simulink model "koen_observer_pll_model"  (R2024b)
settings: Solver=FixedStepDiscrete  StartTime=0.0  StopTime=0.05  FixedStep=6.25e-05  RelTol=1e-3
PreLoadFcn:
  | FOC_TS_SEC=6.25e-05; FOC_RS_OHM=0.53; FOC_LS_H=0.0006; FOC_FLUX_WB=0.0078; FOC_FLUX_LIMIT_RATIO=1.5; FOC_OBS_PLL_KP=180; FOC_OBS_PLL_KI=6000; FOC_OBS_PLL_INTEGRAL_LIMIT=700; FOC_OBS_SPEED_LIMIT_RAD_S=1200; FOC_OBS_SPEED_FILTER_ALPHA=0.2; FOC_OBS_THETA_COMP_RAD=2.7239; FOC_TWO_PI=6.283185307179586;
settings Model: Creator=10095  LastModifiedBy=10095

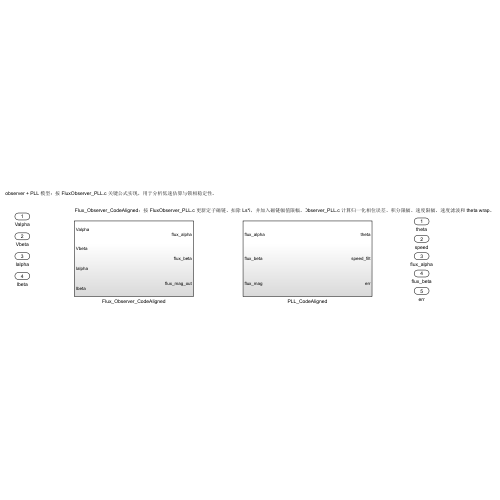
[thumbnail: Simulink's stored preview of the top-level diagram]
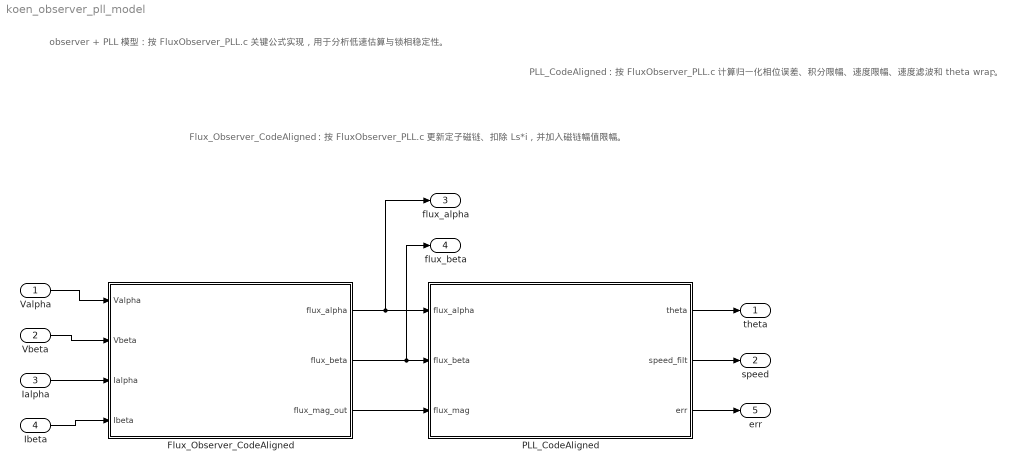
== system koen_observer_pll_model ==
  note: Flux_Observer_CodeAligned：按 FluxObserver_PLL.c 更新定子磁链、扣除 Ls*i，并加入磁链幅值限幅。
  note: PLL_CodeAligned：按 FluxObserver_PLL.c 计算归一化相位误差、积分限幅、速度限幅、速度滤波和 theta wrap。
  note: observer + PLL 模型：按 FluxObserver_PLL.c 关键公式实现，用于分析低速估算与锁相稳定性。
  Valpha : Inport
  Vbeta : Inport  Port=2
  Ialpha : Inport  Port=3
  Ibeta : Inport  Port=4
  Flux_Observer_CodeAligned : Subsystem  Description=Flux_Observer_CodeAligned：按 FluxObserver_PLL.c 更新定子磁链、扣除 Ls*i，并加入磁链幅值限幅。
  PLL_CodeAligned : Subsystem  Description=PLL_CodeAligned：按 FluxObserver_PLL.c 计算归一化相位误差、积分限幅、速度限幅、速度滤波和 theta wrap。
  theta : Outport
  speed : Outport  Port=2
  flux_alpha : Outport  Port=3
  flux_beta : Outport  Port=4
  err : Outport  Port=5
  wires:
  Valpha/1 -> Flux_Observer_CodeAligned/1(Valpha)
  Ialpha/1 -> Flux_Observer_CodeAligned/3(Ialpha)
  Vbeta/1 -> Flux_Observer_CodeAligned/2(Vbeta)
  Ibeta/1 -> Flux_Observer_CodeAligned/4(Ibeta)
  PLL_CodeAligned/1(theta) -> theta/1
  Flux_Observer_CodeAligned/3(flux_mag_out) -> PLL_CodeAligned/3(flux_mag)
  Flux_Observer_CodeAligned/2(flux_beta) -> PLL_CodeAligned/2(flux_beta), flux_beta/1
  PLL_CodeAligned/3(err) -> err/1
  Flux_Observer_CodeAligned/1(flux_alpha) -> flux_alpha/1, PLL_CodeAligned/1(flux_alpha)
  PLL_CodeAligned/2(speed_filt) -> speed/1

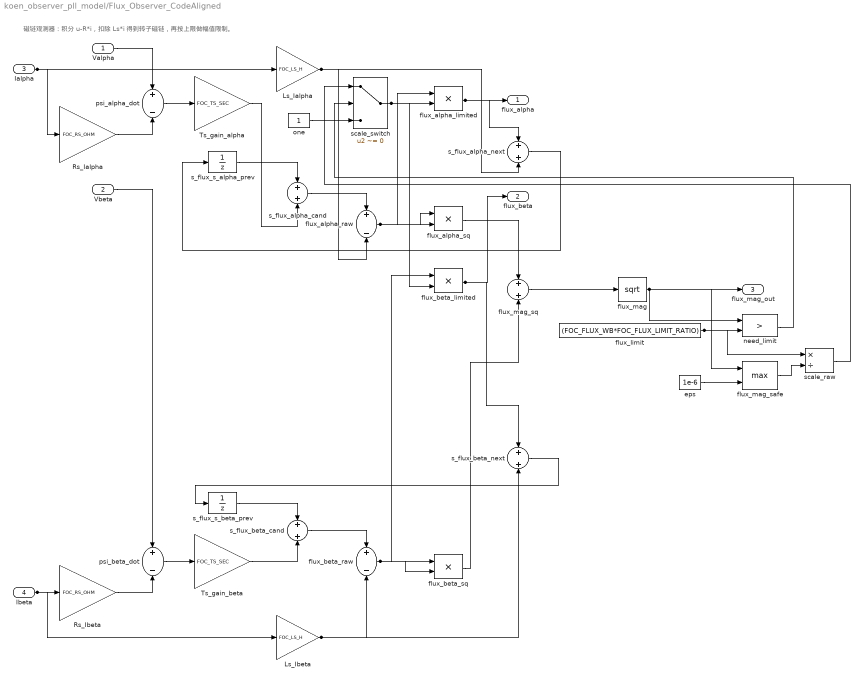
== system koen_observer_pll_model/Flux_Observer_CodeAligned ==
  note: 磁链观测器：积分 u-R*i，扣除 Ls*i 得到转子磁链，再按上限做幅值限制。
  Valpha : Inport
  Vbeta : Inport  Port=2
  Ialpha : Inport  Port=3
  Ibeta : Inport  Port=4
  Ls_Ialpha : Gain  Gain=FOC_LS_H
  Ls_Ibeta : Gain  Gain=FOC_LS_H
  Rs_Ialpha : Gain  Gain=FOC_RS_OHM
  Rs_Ibeta : Gain  Gain=FOC_RS_OHM
  Ts_gain_alpha : Gain  Gain=FOC_TS_SEC
  Ts_gain_beta : Gain  Gain=FOC_TS_SEC
  eps : Constant  Value=1e-6
  flux_alpha_limited : Product
  flux_alpha_raw : Sum  Inputs=+-
  flux_alpha_sq : Product
  flux_beta_limited : Product
  flux_beta_raw : Sum  Inputs=+-
  flux_beta_sq : Product
  flux_limit : Constant  Value=(FOC_FLUX_WB*FOC_FLUX_LIMIT_RATIO)
  flux_mag : Math  Operator=sqrt
  flux_mag_safe : MinMax  Function=max  Inputs=2
  flux_mag_sq : Sum
  need_limit : RelationalOperator  Operator=>  OutDataTypeStr=boolean  RndMeth=Simplest  InputSameDT=off
  one : Constant
  psi_alpha_dot : Sum  Inputs=+-
  psi_beta_dot : Sum  Inputs=+-
  s_flux_alpha_cand : Sum
  s_flux_alpha_next : Sum
  s_flux_beta_cand : Sum
  s_flux_beta_next : Sum
  s_flux_s_alpha_prev : UnitDelay  InitialCondition=FOC_FLUX_WB  SampleTime=FOC_TS_SEC  HasFrameUpgradeWarning=on
  s_flux_s_beta_prev : UnitDelay  SampleTime=FOC_TS_SEC  HasFrameUpgradeWarning=on
  scale_raw : Product  Inputs=*/
  scale_switch : Switch  Criteria=u2 ~= 0  Threshold=0.5  SaturateOnIntegerOverflow=off  InputSameDT=off
  flux_alpha : Outport
  flux_beta : Outport  Port=2
  flux_mag_out : Outport  Port=3
  wires:
  Vbeta/1 -> psi_beta_dot/1
  Ibeta/1 -> Ls_Ibeta/1, Rs_Ibeta/1
  Ialpha/1 -> Ls_Ialpha/1, Rs_Ialpha/1
  s_flux_s_alpha_prev/1 -> s_flux_alpha_cand/1
  Valpha/1 -> psi_alpha_dot/1
  Rs_Ialpha/1 -> psi_alpha_dot/2
  Rs_Ibeta/1 -> psi_beta_dot/2
  psi_alpha_dot/1 -> Ts_gain_alpha/1
  psi_beta_dot/1 -> Ts_gain_beta/1
  Ts_gain_alpha/1 -> s_flux_alpha_cand/2
  flux_limit/1 -> need_limit/2, scale_raw/1
  flux_mag/1 -> need_limit/1, flux_mag_safe/1, flux_mag_out/1
  s_flux_s_beta_prev/1 -> s_flux_beta_cand/1
  Ts_gain_beta/1 -> s_flux_beta_cand/2
  Ls_Ialpha/1 -> flux_alpha_raw/2, s_flux_alpha_next/2
  one/1 -> scale_switch/3
  s_flux_alpha_cand/1 -> flux_alpha_raw/1
  s_flux_alpha_next/1 -> s_flux_s_alpha_prev/1
  flux_alpha_limited/1 -> s_flux_alpha_next/1, flux_alpha/1
  s_flux_beta_cand/1 -> flux_beta_raw/1
  s_flux_beta_next/1 -> s_flux_s_beta_prev/1
  flux_beta_limited/1 -> s_flux_beta_next/1, flux_beta/1
  Ls_Ibeta/1 -> s_flux_beta_next/2, flux_beta_raw/2
  scale_raw/1 -> scale_switch/1
  scale_switch/1 -> flux_alpha_limited/2, flux_beta_limited/2
  flux_alpha_raw/1 -> flux_alpha_sq/1, flux_alpha_sq/2, flux_alpha_limited/1
  flux_beta_raw/1 -> flux_beta_sq/2, flux_beta_limited/1, flux_beta_sq/1
  flux_beta_sq/1 -> flux_mag_sq/2
  flux_alpha_sq/1 -> flux_mag_sq/1
  flux_mag_sq/1 -> flux_mag/1
  eps/1 -> flux_mag_safe/2
  need_limit/1 -> scale_switch/2
  flux_mag_safe/1 -> scale_raw/2

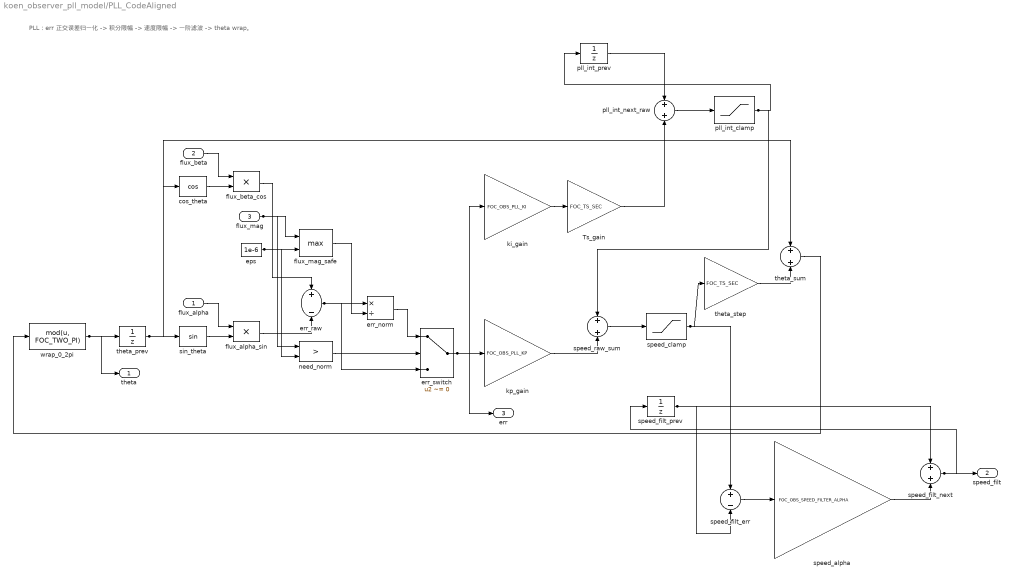
== system koen_observer_pll_model/PLL_CodeAligned ==
  note: PLL：err 正交误差归一化 -> 积分限幅 -> 速度限幅 -> 一阶滤波 -> theta wrap。
  flux_alpha : Inport
  flux_beta : Inport  Port=2
  flux_mag : Inport  Port=3
  Ts_gain : Gain  Gain=FOC_TS_SEC
  cos_theta : Trigonometry  Operator=cos
  eps : Constant  Value=1e-6
  err_norm : Product  Inputs=*/
  err_raw : Sum  Inputs=+-
  err_switch : Switch  Criteria=u2 ~= 0  Threshold=0.5  SaturateOnIntegerOverflow=off  InputSameDT=off
  flux_alpha_sin : Product
  flux_beta_cos : Product
  flux_mag_safe : MinMax  Function=max  Inputs=2
  ki_gain : Gain  Gain=FOC_OBS_PLL_KI
  kp_gain : Gain  Gain=FOC_OBS_PLL_KP
  need_norm : RelationalOperator  Operator=>  OutDataTypeStr=boolean  RndMeth=Simplest  InputSameDT=off
  pll_int_clamp : Saturate  UpperLimit=FOC_OBS_PLL_INTEGRAL_LIMIT  LowerLimit=-FOC_OBS_PLL_INTEGRAL_LIMIT
  pll_int_next_raw : Sum
  pll_int_prev : UnitDelay  SampleTime=FOC_TS_SEC  HasFrameUpgradeWarning=on
  sin_theta : Trigonometry
  speed_alpha : Gain  Gain=FOC_OBS_SPEED_FILTER_ALPHA
  speed_clamp : Saturate  UpperLimit=FOC_OBS_SPEED_LIMIT_RAD_S  LowerLimit=-FOC_OBS_SPEED_LIMIT_RAD_S
  speed_filt_err : Sum  Inputs=+-
  speed_filt_next : Sum
  speed_filt_prev : UnitDelay  SampleTime=FOC_TS_SEC  HasFrameUpgradeWarning=on
  speed_raw_sum : Sum
  theta_prev : UnitDelay  SampleTime=FOC_TS_SEC  HasFrameUpgradeWarning=on
  theta_step : Gain  Gain=FOC_TS_SEC
  theta_sum : Sum
  wrap_0_2pi : Fcn  Expr=mod(u, FOC_TWO_PI)
  theta : Outport
  speed_filt : Outport  Port=2
  err : Outport  Port=3
  wires:
  wrap_0_2pi/1 -> theta_prev/1, theta/1
  theta_prev/1 -> theta_sum/1, sin_theta/1, cos_theta/1
  flux_alpha/1 -> flux_alpha_sin/1
  flux_beta/1 -> flux_beta_cos/1
  err_raw/1 -> err_switch/3, err_norm/1
  flux_beta_cos/1 -> err_raw/1
  sin_theta/1 -> flux_alpha_sin/2
  flux_alpha_sin/1 -> err_raw/2
  cos_theta/1 -> flux_beta_cos/2
  flux_mag/1 -> need_norm/1, flux_mag_safe/1
  need_norm/1 -> err_switch/2
  eps/1 -> need_norm/2, flux_mag_safe/2
  flux_mag_safe/1 -> err_norm/2
  err_norm/1 -> err_switch/1
  err_switch/1 -> ki_gain/1, kp_gain/1, err/1
  ki_gain/1 -> Ts_gain/1
  kp_gain/1 -> speed_raw_sum/2
  pll_int_prev/1 -> pll_int_next_raw/1
  pll_int_clamp/1 -> pll_int_prev/1, speed_raw_sum/1
  Ts_gain/1 -> pll_int_next_raw/2
  speed_raw_sum/1 -> speed_clamp/1
  pll_int_next_raw/1 -> pll_int_clamp/1
  speed_clamp/1 -> speed_filt_err/1, theta_step/1
  speed_filt_prev/1 -> speed_filt_err/2, speed_filt_next/1
  theta_step/1 -> theta_sum/2
  speed_filt_err/1 -> speed_alpha/1
  theta_sum/1 -> wrap_0_2pi/1
  speed_alpha/1 -> speed_filt_next/2
  speed_filt_next/1 -> speed_filt/1, speed_filt_prev/1
